simulink model "px4demo_attitude_control20180822car"  (R2016b)
settings: Solver=FixedStepDiscrete  StartTime=0.0  StopTime=inf  RelTol=1e-3
PostLoadFcn:
  | kFactor = 1.2;
  | 
  | KpRollAttitude = 0.630138625117681 / kFactor;
  | KiRollAttitude = 0.0552303199591522 / kFactor;
  | 
  | KpPitchAttitude = 0.630138625117681 / kFactor;
  | KiPitchAttitude = 0.0552303199591522 / kFactor;
  | 
  | KpRollRate = 1.31533836563383 / kFactor;
  | KiRollRate = 0.460338699849681 / kFactor;
  | 
  | KpPitchRate = 1.31533836563383 / kFactor;
  | KiPitchRate = 0.460338699849681 / kFactor;
  | 
  | KpYawRate = 1.31533836563383 / kFactor;
  | KiYawRate = 0.460338699849681 / kFactor;
libraries: simulink x4
settings Model: Creator=Adam  LastModifiedBy=DELL
settings SolverCC: AutoInsertRateTranBlk=on
settings DataIOCC: LimitDataPoints=on  SaveFormat=Array  SaveOutput=off  SaveTime=off
settings OptimizationCC: BlockReduction=off  DefaultParameterBehavior=Inlined  BufferReuse=off  LifeSpan=1  MaxStackSize=64
settings DebuggingCC: SolverPrmCheckMsg=warning  AllowSymbolicDim=off  SFUnexpectedBacktrackingDiag=warning  SFNoUnconditionalDefaultTransitionDiag=warning  SFExecutionAtInitializationDiag=none
settings HardwareCC: ProdBitPerPointer=32  ProdBitPerSizeT=32  ProdBitPerPtrDiffT=32  ProdLargestAtomicInteger=Long  ProdLargestAtomicFloat=Double  ProdWordSize=32  ProdHWDeviceType=ARM Compatible->ARM Cortex
settings ModelReferenceCC: PropagateSignalLabelsOutOfModel=off
settings RTWCC: SystemTargetFile=ert.tlc  HardwareBoard=Pixhawk PX4  TemplateMakefile=ert_default_tmf  Description=Embedded Coder  GenerateReport=on  Toolchain=Pixhawk Toolchain  IncludeHyperlinkInReport=on  LaunchReport=on  GenerateTraceReport=on  GenerateTraceReportSl=on  GenerateTraceReportSf=on  GenerateTraceReportEml=on  GenerateCodeMetricsReport=on
settings CodeAppCC: IgnoreCustomStorageClasses=off
settings ERTTargetCC: CodeReplacementLibrary=GCC ARM Cortex-A9  SupportContinuousTime=on  ExtModeTransport=1  ExtModeMexFile=ext_serial_win32_comm  ExtModeMexArgs=/dev/serial  ERTCustomFileTemplate=PX4_codertarget_file_process.tlc  ConvertIfToSwitch=off  SuppressUnreachableDefaultCases=off
settings ConfigComp: CovMetricSettings=dw  CovHtmlReporting=on  CovSaveCumulativeToWorkspaceVar=on  CovSaveSingleToWorkspaceVar=on  CovExternalEMLEnable=off  CovSFcnEnable=off

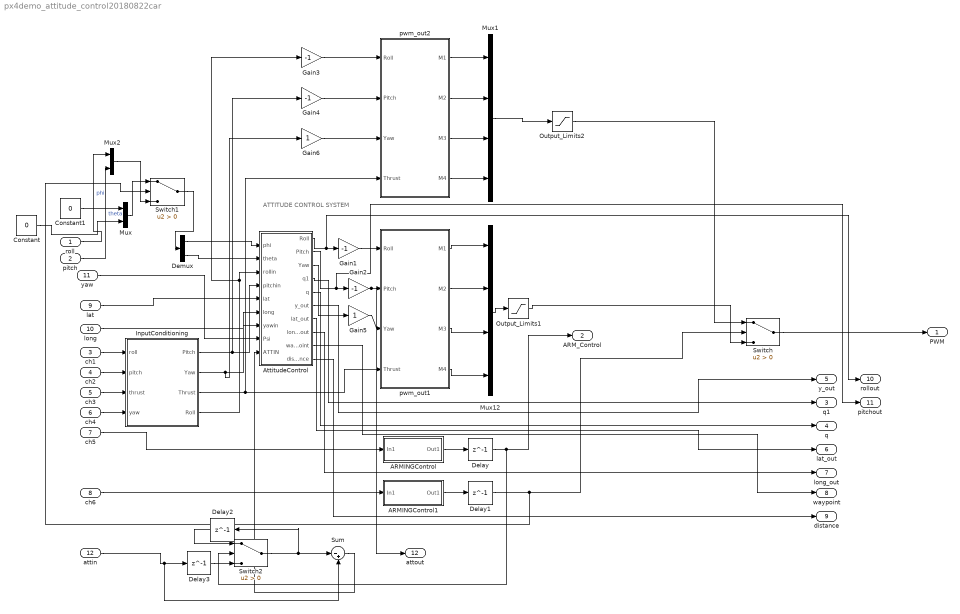
== system px4demo_attitude_control20180822car ==
  note: ATTITUDE CONTROL SYSTEM
  roll : Inport  OutDataTypeStr=single  PortDimensions=1
  pitch : Inport  Port=2  OutDataTypeStr=single  PortDimensions=1
  ch1 : Inport  Port=3  OutDataTypeStr=uint16  PortDimensions=1
  ch2 : Inport  Port=4  OutDataTypeStr=uint16  PortDimensions=1
  ch3 : Inport  Port=5  OutDataTypeStr=uint16  PortDimensions=1
  ch4 : Inport  Port=6  OutDataTypeStr=uint16  PortDimensions=1
  ch5 : Inport  Port=7  OutDataTypeStr=uint16  PortDimensions=1  Interpolate=off
  ch6 : Inport  Port=8  OutDataTypeStr=uint16  PortDimensions=1  Interpolate=off
  lat : Inport  Port=9  OutDataTypeStr=int32  PortDimensions=1  Interpolate=off
  long : Inport  Port=10  OutDataTypeStr=int32  PortDimensions=1  Interpolate=off
  yaw : Inport  Port=11  OutDataTypeStr=single  PortDimensions=1
  attin : Inport  Port=12  OutDataTypeStr=single  PortDimensions=1
  ARMINGControl : Subsystem
  ARMINGControl1 : Subsystem
  AttitudeControl : Subsystem
  Constant : Constant  Value=0  OutDataTypeStr=single
  Constant1 : Constant  Value=0  OutDataTypeStr=single
  Delay{,1..3} (4 alike) : Delay  DelayLength=1  InitialCondition=0
  Demux : Demux  Outputs=2
  Gain{1..4} (4 alike) : Gain  Gain=-1
  Gain5 : Gain
  Gain6 : Gain
  InputConditioning : Subsystem
  Mux : Mux  Inputs=2
  Mux1 : Mux
  Mux12 : Mux
  Mux2 : Mux  Inputs=2
  Output_Limits1 : Saturate  UpperLimit=2000  LowerLimit=1000
  Output_Limits2 : Saturate  UpperLimit=2000  LowerLimit=1000
  Sum : Sum  Inputs=|-+
  Switch : Switch  Criteria=u2 > Threshold
  Switch1 : Switch  Criteria=u2 > Threshold
  Switch2 : Switch  Criteria=u2 > Threshold
  pwm_out1 : MATLAB Function  TreatAsAtomicUnit=on  SystemSampleTime=0.004
  pwm_out2 : MATLAB Function  TreatAsAtomicUnit=on  SystemSampleTime=0.004
  PWM : Outport  PortDimensions=4
  ARM_Control : Outport  Port=2  PortDimensions=1
  q1 : Outport  Port=3
  q : Outport  Port=4
  y_out : Outport  Port=5
  lat_out : Outport  Port=6
  long_out : Outport  Port=7
  waypoint : Outport  Port=8
  distance : Outport  Port=9
  rollout : Outport  Port=10
  pitchout : Outport  Port=11
  attout : Outport  Port=12
  wires:
  Mux12/1 -> Output_Limits1/1
  AttitudeControl/1(Roll) -> rollout/1, Gain1/1
  AttitudeControl/2(Pitch) -> pitchout/1, Gain2/1
  ch5/1 -> ARMINGControl/1(In1)
  pwm_out1/1(M1) -> Mux12/1
  pwm_out1/2(M2) -> Mux12/2
  pwm_out1/3(M3) -> Mux12/3
  pwm_out1/4(M4) -> Mux12/4
  ARMINGControl/1(Out1) -> Delay/1
  Delay/1 -> Switch2/2, ARM_Control/1
  InputConditioning/4(Roll) -> Gain3/1, AttitudeControl/3(rollin)
  InputConditioning/1(Pitch) -> Gain4/1, AttitudeControl/4(pitchin)
  ARMINGControl1/1(Out1) -> Delay1/1
  Delay1/1 -> Switch1/2, Switch/2
  ch6/1 -> ARMINGControl1/1(In1)
  Output_Limits1/1 -> Switch/3
  ch1/1 -> InputConditioning/1(roll)
  ch2/1 -> InputConditioning/2(pitch)
  ch3/1 -> InputConditioning/3(thrust)
  ch4/1 -> InputConditioning/4(yaw)
  Mux1/1 -> Output_Limits2/1
  Gain1/1 -> pwm_out1/1(Roll)
  Switch/1 -> PWM/1
  InputConditioning/3(Thrust) -> pwm_out2/4(Thrust), pwm_out1/4(Thrust)
  InputConditioning/2(Yaw) -> Gain6/1, AttitudeControl/7(yawin)
  AttitudeControl/3(Yaw) -> Gain5/1
  lat/1 -> AttitudeControl/5(lat)
  long/1 -> AttitudeControl/6(long)
  AttitudeControl/4(q1) -> q1/1
  AttitudeControl/5(q) -> q/1
  Output_Limits2/1 -> Switch/1
  pwm_out2/1(M1) -> Mux1/1
  pwm_out2/2(M2) -> Mux1/2
  pwm_out2/3(M3) -> Mux1/3
  pwm_out2/4(M4) -> Mux1/4
  Gain4/1 -> pwm_out2/2(Pitch)
  Gain3/1 -> pwm_out2/1(Roll)
  Gain5/1 -> pwm_out1/3(Yaw)
  Gain6/1 -> pwm_out2/3(Yaw)
  yaw/1 -> AttitudeControl/8(Psi)
  AttitudeControl/6(y_out) -> y_out/1
  AttitudeControl/7(lat_out) -> lat_out/1
  AttitudeControl/8(long_out) -> long_out/1
  AttitudeControl/9(waypoint) -> waypoint/1
  AttitudeControl/10(distance) -> distance/1
  roll/1 -> Mux2/1  "phi"
  pitch/1 -> Mux2/2  "theta"
  Constant1/1 -> Mux/1
  Constant/1 -> Mux/2
  Switch1/1 -> Demux/1
  Demux/1 -> AttitudeControl/1(phi)
  Demux/2 -> AttitudeControl/2(theta)
  Mux/1 -> Switch1/1
  Mux2/1 -> Switch1/3
  Switch2/1 -> Delay2/1, Sum/1
  attin/1 -> Delay3/1, Sum/2
  Sum/1 -> AttitudeControl/9(ATTIN)
  Delay2/1 -> Switch2/1
  Delay3/1 -> Switch2/3
  Gain2/1 -> attout/1, pwm_out1/2(Pitch)

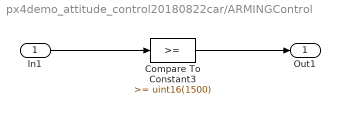
== system px4demo_attitude_control20180822car/ARMINGControl ==
  In1 : Inport
  Compare To Constant3 : simulink/Logic and Bit Operations/Compare To Constant  relop=>=  const=uint16(1500)  OutDataTypeStr=boolean
  Out1 : Outport
  wires:
  Compare To Constant3/1 -> Out1/1
  In1/1 -> Compare To Constant3/1

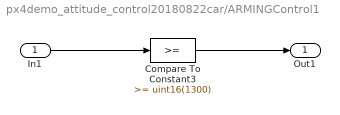
== system px4demo_attitude_control20180822car/ARMINGControl1 ==
  In1 : Inport
  Compare To Constant3 : simulink/Logic and Bit Operations/Compare To Constant  relop=>=  const=uint16(1300)  OutDataTypeStr=boolean
  Out1 : Outport
  wires:
  Compare To Constant3/1 -> Out1/1
  In1/1 -> Compare To Constant3/1

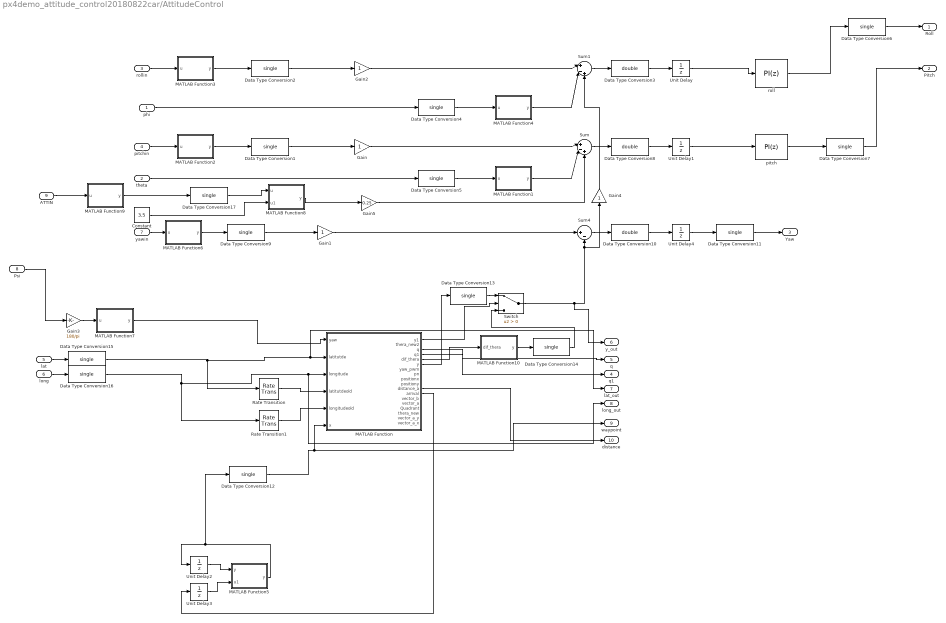
== system px4demo_attitude_control20180822car/AttitudeControl ==
  phi : Inport
  theta : Inport  Port=2
  rollin : Inport  Port=3
  pitchin : Inport  Port=4
  lat : Inport  Port=5
  long : Inport  Port=6
  yawin : Inport  Port=7
  Psi : Inport  Port=8  OutDataTypeStr=single
  ATTIN : Inport  Port=9
  Constant : Constant  Value=3.5
  Data Type Conversion{1..2,4..7,9,11..17} (14 alike) : DataTypeConversion  OutDataTypeStr=single
  Data Type Conversion10 : DataTypeConversion  OutDataTypeStr=double
  Data Type Conversion3 : DataTypeConversion  OutDataTypeStr=double
  Data Type Conversion8 : DataTypeConversion  OutDataTypeStr=double
  Gain{,1..2,4} (4 alike) : Gain
  Gain3 : Gain  Gain=180/pi
  Gain5 : Gain  Gain=0.25
  MATLAB Function : MATLAB Function  TreatAsAtomicUnit=on
  MATLAB Function1 : MATLAB Function  TreatAsAtomicUnit=on
  MATLAB Function10 : MATLAB Function  TreatAsAtomicUnit=on
  MATLAB Function2 : MATLAB Function  TreatAsAtomicUnit=on
  MATLAB Function3 : MATLAB Function  TreatAsAtomicUnit=on
  MATLAB Function4 : MATLAB Function  TreatAsAtomicUnit=on
  MATLAB Function5 : MATLAB Function  TreatAsAtomicUnit=on
  MATLAB Function6 : MATLAB Function  TreatAsAtomicUnit=on
  MATLAB Function7 : MATLAB Function  TreatAsAtomicUnit=on
  MATLAB Function8 : MATLAB Function  TreatAsAtomicUnit=on
  MATLAB Function9 : MATLAB Function  TreatAsAtomicUnit=on
  Rate Transition : RateTransition  OutPortSampleTime=20
  Rate Transition1 : RateTransition  OutPortSampleTime=20
  Sum : Sum  Inputs=|+-+
  Sum1 : Sum  Inputs=|+-+
  Sum4 : Sum  Inputs=|+-
  Switch : Switch  Criteria=u2 > Threshold
  Unit Delay{,1,3..4} (4 alike) : UnitDelay  SampleTime=0.1
  Unit Delay2 : UnitDelay  InitialCondition=1  SampleTime=-1
  pitch : simulink/Continuous/PID Controller  Controller=PI  TimeDomain=Discrete-time  SampleTime=-1  IntegratorMethod=Forward Euler  FilterMethod=Forward Euler  Form=Parallel  UseFilter=on  ControllerParametersSource=internal  P=1.3  I=0.05  D=0.05  N=100  InitialConditionSource=internal  InitialConditionForIntegrator=0  InitialConditionForFilter=0  ExternalReset=none  LimitOutput=on  UpperSaturationLimit=1  LowerSaturationLimit=-1  LinearizeAsGain=on  AntiWindupMode=back-calculation  Kb=1  TrackingMode=off  Kt=1  PParamMin=[]  PParamMax=[]  IParamMin=[]  IParamMax=[]  DParamMin=[]  DParamMax=[]  NParamMin=[]  NParamMax=[]  KbParamMin=[]  KbParamMax=[]  KtParamMin=[]  KtParamMax=[]  POutMin=[]  POutMax=[]  IOutMin=[]  IOutMax=[]  DOutMin=[]  DOutMax=[]  NOutMin=[]  NOutMax=[]  KbOutMin=[]  KbOutMax=[]  KtOutMin=[]  KtOutMax=[]  IntegratorOutMin=[]  IntegratorOutMax=[]  FilterOutMin=[]  FilterOutMax=[]  SumOutMin=[]  SumOutMax=[]  SumI1OutMin=[]  SumI1OutMax=[]  SumI2OutMin=[]  SumI2OutMax=[]  SumI3OutMin=[]  SumI3OutMax=[]  SumDOutMin=[]  SumDOutMax=[]  SaturationOutMin=[]  SaturationOutMax=[]  IntegratorContinuousStateAttributes=''  IntegratorStateMustResolveToSignalObject=off  IntegratorRTWStateStorageClass=Auto  FilterContinuousStateAttributes=''  FilterStateMustResolveToSignalObject=off  FilterRTWStateStorageClass=Auto  DifferentiatorICPrevScaledInput=0  DifferentiatorOutMin=[]  DifferentiatorOutMax=[]
  roll : simulink/Continuous/PID Controller  Controller=PI  TimeDomain=Discrete-time  SampleTime=-1  IntegratorMethod=Forward Euler  FilterMethod=Forward Euler  Form=Parallel  UseFilter=on  ControllerParametersSource=internal  P=1  I=0.05  D=0.1  N=100  InitialConditionSource=internal  InitialConditionForIntegrator=0  InitialConditionForFilter=0  ExternalReset=none  LimitOutput=on  UpperSaturationLimit=1  LowerSaturationLimit=-1  LinearizeAsGain=on  AntiWindupMode=back-calculation  Kb=1  TrackingMode=off  Kt=1  PParamMin=[]  PParamMax=[]  IParamMin=[]  IParamMax=[]  DParamMin=[]  DParamMax=[]  NParamMin=[]  NParamMax=[]  KbParamMin=[]  KbParamMax=[]  KtParamMin=[]  KtParamMax=[]  POutMin=[]  POutMax=[]  IOutMin=[]  IOutMax=[]  DOutMin=[]  DOutMax=[]  NOutMin=[]  NOutMax=[]  KbOutMin=[]  KbOutMax=[]  KtOutMin=[]  KtOutMax=[]  IntegratorOutMin=[]  IntegratorOutMax=[]  FilterOutMin=[]  FilterOutMax=[]  SumOutMin=[]  SumOutMax=[]  SumI1OutMin=[]  SumI1OutMax=[]  SumI2OutMin=[]  SumI2OutMax=[]  SumI3OutMin=[]  SumI3OutMax=[]  SumDOutMin=[]  SumDOutMax=[]  SaturationOutMin=[]  SaturationOutMax=[]  IntegratorContinuousStateAttributes=''  IntegratorStateMustResolveToSignalObject=off  IntegratorRTWStateStorageClass=Auto  FilterContinuousStateAttributes=''  FilterStateMustResolveToSignalObject=off  FilterRTWStateStorageClass=Auto  DifferentiatorICPrevScaledInput=0  DifferentiatorOutMin=[]  DifferentiatorOutMax=[]
  Roll : Outport
  Pitch : Outport  Port=2
  Yaw : Outport  Port=3
  q1 : Outport  Port=4
  q : Outport  Port=5
  y_out : Outport  Port=6
  lat_out : Outport  Port=7
  long_out : Outport  Port=8
  waypoint : Outport  Port=9
  distance : Outport  Port=10
  wires:
  Gain/1 -> Sum/1
  Gain2/1 -> Sum1/1
  rollin/1 -> MATLAB Function3/1(u)
  pitchin/1 -> MATLAB Function2/1(u)
  theta/1 -> Data Type Conversion5/1
  Sum/1 -> Data Type Conversion8/1
  Sum1/1 -> Data Type Conversion3/1
  pitch/1 -> Data Type Conversion7/1
  roll/1 -> Data Type Conversion6/1
  Data Type Conversion5/1 -> MATLAB Function1/1(u)
  Data Type Conversion4/1 -> MATLAB Function4/1(u)
  Data Type Conversion6/1 -> Roll/1
  Data Type Conversion7/1 -> Pitch/1
  MATLAB Function4/1(y) -> Sum1/2
  MATLAB Function1/1(y) -> Sum/2
  MATLAB Function3/1(y) -> Data Type Conversion2/1
  Data Type Conversion2/1 -> Gain2/1
  phi/1 -> Data Type Conversion4/1
  Unit Delay/1 -> roll/1
  Unit Delay1/1 -> pitch/1
  Data Type Conversion3/1 -> Unit Delay/1
  Data Type Conversion8/1 -> Unit Delay1/1
  lat/1 -> Data Type Conversion15/1
  long/1 -> Data Type Conversion16/1
  Unit Delay2/1 -> MATLAB Function5/1("y ")
  MATLAB Function5/1(y) -> Data Type Conversion12/1, Unit Delay2/1
  Unit Delay3/1 -> MATLAB Function5/2(u1)
  MATLAB Function/12(arrival) -> Unit Delay3/1
  MATLAB Function2/1(y) -> Data Type Conversion1/1
  Data Type Conversion1/1 -> Gain/1
  yawin/1 -> MATLAB Function6/1(u)
  MATLAB Function6/1(y) -> Data Type Conversion9/1
  Data Type Conversion9/1 -> Gain1/1
  Gain1/1 -> Sum4/1
  MATLAB Function10/1(y) -> Data Type Conversion14/1
  Sum4/1 -> Data Type Conversion10/1
  Data Type Conversion10/1 -> Unit Delay4/1
  Unit Delay4/1 -> Data Type Conversion11/1
  Data Type Conversion11/1 -> Yaw/1
  Data Type Conversion12/1 -> waypoint/1, MATLAB Function/6(x)
  Data Type Conversion14/1 -> Switch/3
  Rate Transition/1 -> MATLAB Function/4(latitutdeold)
  Rate Transition1/1 -> MATLAB Function/5(longitudeold)
  MATLAB Function7/1(y) -> MATLAB Function/1(yaw)
  MATLAB Function/5(dif_thera) -> MATLAB Function10/1(dif_thera)
  MATLAB Function/1(y1) -> Switch/2
  MATLAB Function/6(y) -> Data Type Conversion13/1
  Switch/1 -> Gain4/1, Sum4/2, y_out/1
  Data Type Conversion13/1 -> Switch/1
  Gain3/1 -> MATLAB Function7/1(u)
  Psi/1 -> Gain3/1
  Data Type Conversion15/1 -> lat_out/1, MATLAB Function/2(latitutde), Rate Transition/1
  Data Type Conversion16/1 -> long_out/1, MATLAB Function/3(longitude), Rate Transition1/1
  MATLAB Function/3(q) -> q/1
  MATLAB Function/4(q1) -> q1/1
  MATLAB Function/11(distance_a) -> distance/1
  Gain4/1 -> Sum1/3
  ATTIN/1 -> MATLAB Function9/1(u)
  Data Type Conversion17/1 -> MATLAB Function8/1(u)
  MATLAB Function8/1(y) -> Gain5/1
  Constant/1 -> MATLAB Function8/2(u1)
  Gain5/1 -> Sum/3
  MATLAB Function9/1(y) -> Data Type Conversion17/1

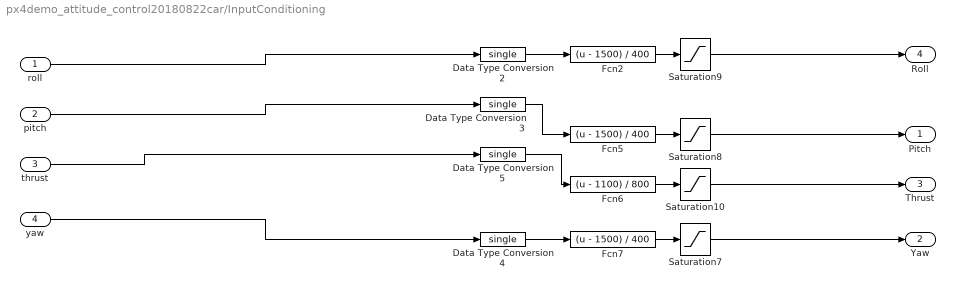
== system px4demo_attitude_control20180822car/InputConditioning ==
  roll : Inport
  pitch : Inport  Port=2
  thrust : Inport  Port=3
  yaw : Inport  Port=4
  Data Type Conversion{2..5} (4 alike) : DataTypeConversion  OutDataTypeStr=single
  Fcn2 : Fcn  Expr=(u - 1500) / 400
  Fcn5 : Fcn  Expr=(u - 1500) / 400
  Fcn6 : Fcn  Expr=(u - 1100) / 800
  Fcn7 : Fcn  Expr=(u - 1500) / 400
  Saturation10 : Saturate  UpperLimit=1  LowerLimit=0
  Saturation7 : Saturate  UpperLimit=1  LowerLimit=-1
  Saturation8 : Saturate  UpperLimit=1  LowerLimit=-1
  Saturation9 : Saturate  UpperLimit=1  LowerLimit=-1
  Pitch : Outport
  Yaw : Outport  Port=2
  Thrust : Outport  Port=3
  Roll : Outport  Port=4
  wires:
  Fcn6/1 -> Saturation10/1
  thrust/1 -> Data Type Conversion5/1
  Fcn2/1 -> Saturation9/1
  Fcn5/1 -> Saturation8/1
  Fcn7/1 -> Saturation7/1
  yaw/1 -> Data Type Conversion4/1
  pitch/1 -> Data Type Conversion3/1
  Data Type Conversion2/1 -> Fcn2/1
  Data Type Conversion3/1 -> Fcn5/1
  Data Type Conversion4/1 -> Fcn7/1
  Data Type Conversion5/1 -> Fcn6/1
  roll/1 -> Data Type Conversion2/1
  Saturation8/1 -> Pitch/1
  Saturation7/1 -> Yaw/1
  Saturation10/1 -> Thrust/1
  Saturation9/1 -> Roll/1

== matlab function px4demo_attitude_control20180822car/AttitudeControl/MATLAB Function1 ==
  data: u input; y output
function y = fcn(u)

y = round(u*10)/10;

== matlab function px4demo_attitude_control20180822car/AttitudeControl/MATLAB Function ==
  data: yaw input; y1 output; thera_new2 output; q output; q1 output; dif_thera output; y output; latitutde input; yaw_pwm output; longitude input; latitutdeold input; longitudeold input; x input; pn output; positionx output; positiony output; distance_a output; arrival output; vector_b output; vector_a output; Quadrant output; thera_new output; vector_a_y output; vector_a_x output
function [y1,thera_new2,q,q1,dif_thera,y,yaw_pwm,pn,positionx,positiony,distance_a,arrival,vector_b,vector_a,Quadrant,thera_new,vector_a_y,vector_a_x]  = fcn(yaw,latitutde,longitude,latitutdeold,longitudeold,x)
position=[251981990,1214213880;
          251989590,1214219020;]
          

yaw_pwm=0
thera_new=0
vector_a=[(position(x,1)-latitutde),(position(x,2)-longitude)]
vector_a_y=(position(x,1)-latitutde)
vector_a_x=(position(x,2)-longitude)
vector_b=[(latitutdeold-latitutde),(longitudeold-longitude)]
distance_a=sqrt((position(x,1)-latitutde)^2+(position(x,2)-longitude)^2)
distance_b=sqrt((latitutdeold-latitutde)^2+(longitudeold-longitude)^2+0.0000001)
%thera=acosd(dot(vector_a,vector_b)/(distance_a*distance_b))
%thera_new=acosd(dot(vector_a,vector_b)/(distance_a*distance_b))
thera_new1=atand(vector_a_y/vector_a_x)
vector_a1=[(position(x,1)-latitutde),(position(x,2)-longitude),0]
vector_b1=[(latitutdeold-latitutde),(longitudeold-longitude),0]
vector_b1_new=[1,0,0]
distance_a=distance_a/1000;

%vector_a_y=(position(x,1)-latitutde);
%vector_a_x=(position(x,2)-longitude);
thera_new2=atand(vector_a_x/vector_a_y);

if(position(x,1)>=latitutde && position(x,2) >= longitude)
    thera_new2=abs(thera_new2)
    q=1
elseif(position(x,1)<=latitutde && position(x,2) >= longitude)
    thera_new2=90+(thera_new2+90)
    q=2
    elseif(position(x,1)<=latitutde && position(x,2) <= longitude)
        thera_new2=180+thera_new2
       q=3 
else
    thera_new2=270+(thera_new2+90)
    q=4
end
if(yaw <=90 && yaw>0 )
    q1=1
elseif(yaw <=180 && yaw>90)
    q1=2
elseif(yaw<=270 && yaw>180)
    q1=3
else
    q1=4
end
dif_thera=thera_new2-yaw;
if(q==4 && q1==1)
    y=-0.4
    y1=1
elseif(q==4 && q1==2)
    y=-1
    y1=1
elseif(q==4 && q1==3)
    y=0.4
    y1=1
    %
elseif(q==3 && q1==4)
    y=-0.4
    y1=1
elseif(q==3 && q1==1)
    y=-1
    y1=1
elseif(q==3 && q1==2)
    y=0.4
    y1=1
    %
elseif(q==2 && q1==4)
    y=-1
    y1=1
elseif(q==2 && q1==1)
    y=0.4
    y1=1
elseif(q==2 && q1==3)
    y=-0.4
    y1=1
     %
elseif(q==1 && q1==4)
    y=0.4
    y1=1
elseif(q==1 && q1==2)
    y=-0.4
    y1=1
elseif(q==1 && q1==3)
    y=-1
    y1=1
elseif(q==q1)
    y1=0
    y=0
    
elseif(thera_new2 == 90)
     y=0
     y1=1
elseif(thera_new2 == 180)
     y=0
     y1=1
elseif(thera_new2 == 270)
     y=0
     y1=1
elseif(thera_new2 == 270)
     y=0
     y1=1
%elseif(q==q1 & dif_thera <79 & dif_thera>=69)
%    y=0.8
%elseif(q==q1 & dif_thera <69 & dif_thera>=59)
%    y=0.7
%elseif(q==q1 & dif_thera <59 & dif_thera>=49)
%    y=0.6
%elseif(q==q1 & dif_thera <49 & dif_thera>=39)
%    y=0.5
%elseif(q==q1 & dif_thera <39 & dif_thera>=29)
%    y=0.4
%elseif(q==q1 & dif_thera <29 & dif_thera>=19)
%    y=0.3
%elseif(q==q1 & dif_thera <19 & dif_thera>=9)
 %   y=0.2
%elseif(q==q1 & dif_thera <9 & dif_thera >=0)
 %   y=0
    %
%elseif(q==q1 & dif_thera <-89 & dif_thera>=-79)
%    y=-0.9
%elseif(q==q1 & dif_thera <-79 & dif_thera>=-69)
%    y=-0.8
%elseif(q==q1 & dif_thera <-69 & dif_thera>=-59)
%    y=-0.7
%elseif(q==q1 & dif_thera <-59 & dif_thera>=-49)
%    y=-0.6
%elseif(q==q1 & dif_thera <-49 & dif_thera>=-39)
%    y=-0.5
%elseif(q==q1 & dif_thera <-39 & dif_thera>=-29)
%    y=-0.4
%elseif(q==q1 & dif_thera <-29 & dif_thera>=-19)
%    y=-0.3
%elseif(q==q1 & dif_thera <-19 & dif_thera>=-9)
%    y=-0.2
%elseif(q==q1 & dif_thera <-9 & dif_thera > 0)
%    y=-0
else
    y=0.
    y1=1
end
%dif_thera=thera_new2-yaw;

%if(vector_a_y>=0 && vector_a_x >=0)
%    thera_new1=abs(thera_new1)
%elseif(vector_a_y>=0 && vector_a_x <=0)
%    thera_new1=thera_new1+90
%    elseif(vector_a_y<=0 && vector_a_x <=0)
%    thera_new1=thera_new1+180
%    elseif(vector_a_y<=0 && vector_a_x >=0)
%    thera_new1=thera_new1+270
%end
%dif_thera=(thera_new1-yaw)+360
%if(dif_thera>=360)
%    dif_thera=dif_thera-360
%end








pn=cross(vector_a1,vector_b1)
pn_new=cross(vector_a1,vector_b1)
positionx=position(x,1)
positiony=position(x,2)

%if((latitutdeold-latitutde)==0 && (longitudeold-longitude)==0 )
%yaw_pwm=single(180)
%elseif(pn(1,3)>0)
% yaw_pwm=-(single(thera))
%else
 %yaw_pwm=single(thera)
%end

if(abs(position(x,1)) > abs(latitutde) && abs(position(x,2)) < abs(longitude))
Quadrant=1
elseif(abs(position(x,1)) > abs(latitutde) && abs(position(x,2)) > abs(longitude))
Quadrant=2
elseif(abs(position(x,1)) < abs(latitutde) && abs(position(x,2)) > abs(longitude))
Quadrant=3
elseif(abs(position(x,1)) < abs(latitutde) && abs(position(x,2)) < abs(longitude))
Quadrant=4
else
    Quadrant=0
end
if(distance_a < 2 )
   arrival=round(1)
else
    arrival=round(0)
end
%&& distance_a > 0.002
%if(x == 3 && distance_a < 0.08) 
% reset=round(-3)
%else
 % reset=round(0)
%end

== matlab function px4demo_attitude_control20180822car/AttitudeControl/MATLAB Function3 ==
  data: u input; y output
function y = fcn(u)

y = round(u*100)/100;

== matlab function px4demo_attitude_control20180822car/pwm_out1 ==
  data: Roll input; M1 output; Pitch input; Yaw input; Thrust input; M2 output; M3 output; M4 output
function [M1, M2, M3, M4] = motor_mixer(Roll, Pitch, Yaw, Thrust)

%idle_PWM = uint16(1000);

% Quad X
% M1 = ((Roll + Pitch - Yaw) / 2 * Thrust + Thrust) * 1000 + idle_PWM;
% M2 = ((-Roll + Pitch + Yaw) / 2 * Thrust + Thrust) * 1000 + idle_PWM;
% M3 = ((-Roll - Pitch - Yaw) / 2 * Thrust + Thrust) * 1000 + idle_PWM;
% M4 = ((Roll - Pitch + Yaw) / 2 * Thrust + Thrust) * 1000 + idle_PWM;
% M5 = 1000;
% M6 = 1000;
% M7 = 1000;
% M8 = 1000;

% Quad +
% M1 = ((Pitch - Yaw) * Thrust / 2 + Thrust) * 1000 + idle_PWM;
% M2 = ((-Roll + Yaw) * Thrust / 2 + Thrust) * 1000 + idle_PWM;
% M3 = ((-Pitch - Yaw) * Thrust / 2 + Thrust) * 1000 + idle_PWM;
% M4 = ((Roll + Yaw) * Thrust / 2 + Thrust) * 1000 + idle_PWM;
% M5 = 1000;
% M6 = 1000;
% M7 = 1000;
% M8 = 1000;

% Hex X
% M1 = ((Pitch + Roll / 2 - Yaw) * Thrust / 2 + Thrust) * 1000 + idle_PWM;
% M2 = ((Pitch - Roll / 2 + Yaw) * Thrust / 2 + Thrust) * 1000 + idle_PWM;
% M3 = ((-Roll - Yaw) * Thrust / 2 + Thrust) * 1000 + idle_PWM;
% M4 = ((-Pitch - Roll / 2 + Yaw) * Thrust / 2 + Thrust) * 1000 + idle_PWM;
% M5 = ((-Pitch + Roll / 2 - Yaw) * Thrust / 2 + Thrust) * 1000 + idle_PWM;
% M6 = ((Roll + Yaw) * Thrust / 2 + Thrust) * 1000 + idle_PWM;
% M7 = 1000;
% M8 = 1000;

% Hex X (From Adam)
M1 = uint16(single(1500+(Roll)*400));
M2 = uint16(single(1500+(Pitch)*400));
M3 = uint16(single(1100+(Thrust)*800));
M4 = uint16(single(1500+(Yaw)*400));


% Hex X (Version 2)
% Roll/Yaw
% M1 = ((-Roll - Yaw) * Thrust / 2 + Thrust) * 1000 + idle_PWM;
% M2 = ((Roll + Yaw) * Thrust / 2 + Thrust) * 1000 + idle_PWM;
% % + Pitch/Roll
% M6 = ((Pitch + Roll / 2 - Yaw) * Thrust / 2 + Thrust) * 1000 + idle_PWM;
% M4 = ((Pitch - Roll / 2 + Yaw) * Thrust / 2 + Thrust) * 1000 + idle_PWM;
% % - Pitch/Roll
% M5 = ((-Pitch - Roll / 2 + Yaw) * Thrust / 2 + Thrust) * 1000 + idle_PWM;
% M3 = ((-Pitch + Roll / 2 - Yaw) * Thrust / 2 + Thrust) * 1000 + idle_PWM;

== matlab function px4demo_attitude_control20180822car/AttitudeControl/MATLAB Function2 ==
  data: u input; y output
function y = fcn(u)

y = round(u*100)/100;

== matlab function px4demo_attitude_control20180822car/AttitudeControl/MATLAB Function4 ==
  data: u input; y output
function y = fcn(u)

y = round(u*10)/10;

== matlab function px4demo_attitude_control20180822car/AttitudeControl/MATLAB Function5 ==
  data: y input; y output; u1 input
function y = fcn(y,u1)
if(u1 == 1 && y <= 3)
y = y+1;
end
if(y == 3)
y=1;
end

== matlab function px4demo_attitude_control20180822car/AttitudeControl/MATLAB Function6 ==
  data: u input; y output
function y = fcn(u)

y = round(u*100)/100;

== matlab function px4demo_attitude_control20180822car/AttitudeControl/MATLAB Function7 ==
  data: u input; y output
function y = fcn(u)
if(u<=0)
    y=360+u;
else
    y=u
end

== matlab function px4demo_attitude_control20180822car/pwm_out2 ==
  data: Roll input; M1 output; Pitch input; Yaw input; Thrust input; M2 output; M3 output; M4 output
function [M1, M2, M3, M4] = motor_mixer(Roll, Pitch, Yaw, Thrust)

%idle_PWM = uint16(1000);

% Quad X
% M1 = ((Roll + Pitch - Yaw) / 2 * Thrust + Thrust) * 1000 + idle_PWM;
% M2 = ((-Roll + Pitch + Yaw) / 2 * Thrust + Thrust) * 1000 + idle_PWM;
% M3 = ((-Roll - Pitch - Yaw) / 2 * Thrust + Thrust) * 1000 + idle_PWM;
% M4 = ((Roll - Pitch + Yaw) / 2 * Thrust + Thrust) * 1000 + idle_PWM;
% M5 = 1000;
% M6 = 1000;
% M7 = 1000;
% M8 = 1000;

% Quad +
% M1 = ((Pitch - Yaw) * Thrust / 2 + Thrust) * 1000 + idle_PWM;
% M2 = ((-Roll + Yaw) * Thrust / 2 + Thrust) * 1000 + idle_PWM;
% M3 = ((-Pitch - Yaw) * Thrust / 2 + Thrust) * 1000 + idle_PWM;
% M4 = ((Roll + Yaw) * Thrust / 2 + Thrust) * 1000 + idle_PWM;
% M5 = 1000;
% M6 = 1000;
% M7 = 1000;
% M8 = 1000;

% Hex X
% M1 = ((Pitch + Roll / 2 - Yaw) * Thrust / 2 + Thrust) * 1000 + idle_PWM;
% M2 = ((Pitch - Roll / 2 + Yaw) * Thrust / 2 + Thrust) * 1000 + idle_PWM;
% M3 = ((-Roll - Yaw) * Thrust / 2 + Thrust) * 1000 + idle_PWM;
% M4 = ((-Pitch - Roll / 2 + Yaw) * Thrust / 2 + Thrust) * 1000 + idle_PWM;
% M5 = ((-Pitch + Roll / 2 - Yaw) * Thrust / 2 + Thrust) * 1000 + idle_PWM;
% M6 = ((Roll + Yaw) * Thrust / 2 + Thrust) * 1000 + idle_PWM;
% M7 = 1000;
% M8 = 1000;

% Hex X (From Adam)
M1 = uint16(single(1500+(Roll)*400));
M2 = uint16(single(1500+(Pitch)*400));
M3 = uint16(single(1100+(Thrust)*800));
M4 = uint16(single(1500+(Yaw)*400));


% Hex X (Version 2)
% Roll/Yaw
% M1 = ((-Roll - Yaw) * Thrust / 2 + Thrust) * 1000 + idle_PWM;
% M2 = ((Roll + Yaw) * Thrust / 2 + Thrust) * 1000 + idle_PWM;
% % + Pitch/Roll
% M6 = ((Pitch + Roll / 2 - Yaw) * Thrust / 2 + Thrust) * 1000 + idle_PWM;
% M4 = ((Pitch - Roll / 2 + Yaw) * Thrust / 2 + Thrust) * 1000 + idle_PWM;
% % - Pitch/Roll
% M5 = ((-Pitch - Roll / 2 + Yaw) * Thrust / 2 + Thrust) * 1000 + idle_PWM;
% M3 = ((-Pitch + Roll / 2 - Yaw) * Thrust / 2 + Thrust) * 1000 + idle_PWM;

== matlab function px4demo_attitude_control20180822car/AttitudeControl/MATLAB Function8 ==
  data: u input; y output; u1 input
function y = fcn(u,u1)
u2=u1+2;
u3=u1-2;
if(u<=u3)
    y=1;
elseif(u>=u2)
    y=-1;
else
    y=0;
    
end

== matlab function px4demo_attitude_control20180822car/AttitudeControl/MATLAB Function9 ==
  data: u input; y output
function y = fcn(u)

y = round(u);

== matlab function px4demo_attitude_control20180822car/AttitudeControl/MATLAB Function10 ==
  data: dif_thera input; y output
function y = fcn(dif_thera)

if(dif_thera <89 & dif_thera>=79)
    y=0.9
elseif(dif_thera <79 & dif_thera>=69)
    y=0.8
elseif(dif_thera <69 & dif_thera>=59)
    y=0.7
elseif(dif_thera <59 & dif_thera>=49)
    y=0.6
elseif(dif_thera <49 & dif_thera>=39)
    y=0.5
elseif(dif_thera <39 & dif_thera>=29)
    y=0.4
elseif(dif_thera <29 & dif_thera>=19)
    y=0.3
elseif(dif_thera <19 & dif_thera>=9)
    y=0.2
elseif(dif_thera <9 & dif_thera >=0)
    y=0
    %
elseif(dif_thera >-89 & dif_thera<=-79)
    y=-0.9
elseif(dif_thera >-79 & dif_thera<=-69)
    y=-0.8
elseif(dif_thera >-69 & dif_thera<=-59)
    y=-0.7
elseif(dif_thera >-59 & dif_thera<=-49)
    y=-0.6
elseif(dif_thera >-49 & dif_thera<=-39)
    y=-0.5
elseif(dif_thera >-39 & dif_thera<=-29)
    y=-0.4
elseif(dif_thera >-29 & dif_thera<=-19)
    y=-0.3
elseif(dif_thera >-19 & dif_thera<=-9)
    y=-0.2
elseif(dif_thera >-9 & dif_thera < 0)
    y=-0
else
    y=0
end
